simulink model "Aircraft_Simulator_full_long"  (R2024b)
settings: Solver=ode4  StartTime=0.0  StopTime=tfinal  FixedStep=dt  RelTol=1e-3
values from neighbouring files (symbols this model uses):
  A = [Xu  Xw  -w0  -9.81*cos(theta0) ... (first row only)    [Task3_code.m]
  A_long_period = [Xu+(w0*Zu)/(Zq+u0) -9.81*cos(theta0)-(w0*9.81*sin(theta0)/(Zq+u0)) ... (first row only)    [Task3_code.m]
  A_short_period = [Zw/(1-Zwd), (Zq+u0)/(1-Zwd) ... (first row only)    [Task3_code.m]
  aircraft_data = xlsread(filename_density_L, 'B2:B61')    [Task3_code.m]
  B = [Xde  Xdth ... (first row only)    [Task3_code.m]
  B_long_period = [Xde+(w0*Zde)/(Zq+u0) Xdth+(w0*Zdth)/(Zq+u0) ... (first row only)    [Task3_code.m]
  B_short_period = [Zde/(1-Zwd), Zdth/(1-Zwd) ... (first row only)    [Task3_code.m]
  C = eye(4,4)    [Task3_code.m]
  D = zeros(4,2)    [Task3_code.m]
  da = dc(1)    [Task3_code.m]
  de = 0    [Task3_code.m]
  dr = dc(2)    [Task3_code.m]
  dth = 10000    [Task3_code.m]
  F_gravity_0 = m*g * [ sin(s0(8)) ... (first row only)    [Task3_code.m]
  initial_conditions = [aircraft_data(13:15)' aircraft_data(10:12)' aircraft_data(4:6)' aircraft_data(7:9)' aircraft_data(18) aircraft_data(20) Vto 0]    [Task3_code.m]
  Ixx = aircraft_data(53)    [Task3_code.m]
  Iyy = aircraft_data(54)    [Task3_code.m]
  Izz = aircraft_data(55)    [Task3_code.m]
  m = aircraft_data(51)    [Task3_code.m]
  M0 = [0; 0; 0]    [Task3_code.m]
  s0 = aircraft_data(4:15)    [Task3_code.m]
undefined symbols (not defined in the file or in its folder): Matrix_Controls, Matrix_states
libraries: simulink_extras x8, shared6dof x1, aerolibasang x1
settings Model: Creator=yossef  LastModifiedBy=sheri
settings SolverCC: AlgebraicLoopSolver=TrustRegion
settings DataIOCC: ReturnWorkspaceOutputs=off
settings DebuggingCC: UnconnectedInputMsg=warning  UnconnectedOutputMsg=warning  UnconnectedLineMsg=warning  ArithmeticOperatorsInVariantConditions=warning
settings ModelReferenceCC: EnableRefExpFcnMdlSchedulingChecks=on
settings SFSimCC: SimUseLocalCustomCode=off  CustomCodeUndefinedFunction=UseInterfaceOnly
settings RTWCC: RTWUseLocalCustomCode=off  GPUComputeCapability=3.5

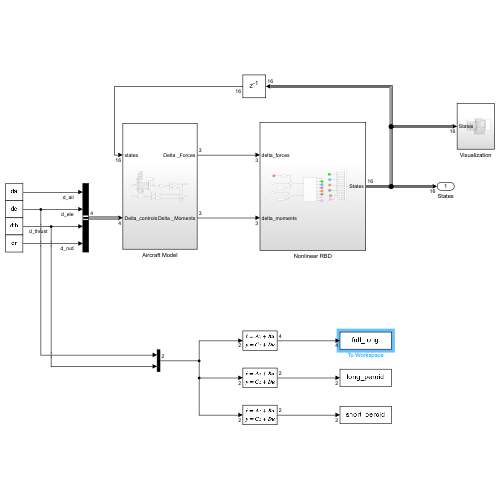
[thumbnail: Simulink's stored preview of the top-level diagram]
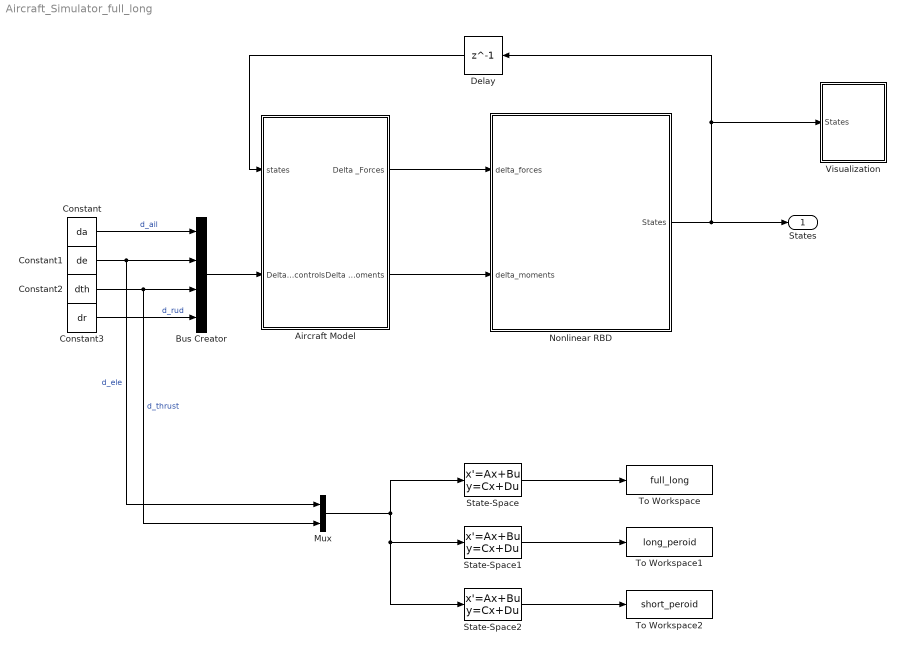
== system Aircraft_Simulator_full_long ==
  Aircraft Model : Subsystem
  Bus Creator : BusCreator  Inputs=4
  Constant : Constant  Value=da
  Constant1 : Constant  Value=de
  Constant2 : Constant  Value=dth
  Constant3 : Constant  Value=dr
  Delay : Delay  DelayLength=1  InitialCondition=initial_conditions
  Mux : Mux  Inputs=2
  Nonlinear RBD : Subsystem
  State-Space : StateSpace  A=A  B=B  C=C  D=D  InitialCondition=[s0(1),s0(3),s0(5),s0(8)]
  State-Space1 : StateSpace  A=A_long_period  B=B_long_period  C=eye(2,2)  D=zeros(2,2)  InitialCondition=[s0(1),s0(8)]
  State-Space2 : StateSpace  A=A_short_period  B=B_short_period  C=eye(2,2)  D=zeros(2,2)  InitialCondition=[aircraft_data(18),s0(5)]
  To Workspace : ToWorkspace  VariableName=full_long  SaveFormat=Timeseries  SampleTime=-1
  To Workspace1 : ToWorkspace  VariableName=long_peroid  SaveFormat=Timeseries  SampleTime=-1
  To Workspace2 : ToWorkspace  VariableName=short_peroid  SaveFormat=Timeseries  SampleTime=-1
  Visualization : Subsystem
  States : Outport
  wires:
  Delay/1 -> Aircraft Model/1(states)
  Nonlinear RBD/1(States) -> States/1, Delay/1, Visualization/1(States)
  Aircraft Model/1(Delta _Forces) -> Nonlinear RBD/1(delta_forces)
  Aircraft Model/2(Delta _Moments) -> Nonlinear RBD/2(delta_moments)
  Constant/1 -> Bus Creator/1  "d_ail"
  Constant1/1 -> Mux/1, Bus Creator/2  "d_ele"
  Constant2/1 -> Mux/2, Bus Creator/3  "d_thrust"
  Constant3/1 -> Bus Creator/4  "d_rud"
  Bus Creator/1 -> Aircraft Model/2(Delta_controls)
  Mux/1 -> State-Space/1, State-Space2/1, State-Space1/1
  State-Space/1 -> To Workspace/1
  State-Space2/1 -> To Workspace2/1
  State-Space1/1 -> To Workspace1/1

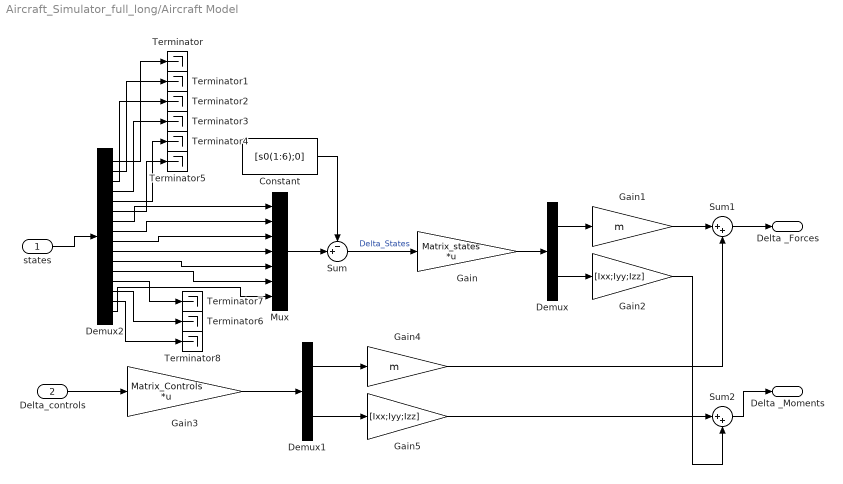
== system Aircraft_Simulator_full_long/Aircraft Model ==
  states : Inport
  Delta_controls : Inport  Port=2
  Constant : Constant  Value=[s0(1:6);0]
  Demux : Demux  Outputs=2
  Demux1 : Demux  Outputs=2
  Demux2 : Demux  Outputs=16
  Gain : Gain  Gain=Matrix_states  Multiplication=Matrix(K*u)
  Gain1 : Gain  Gain=m
  Gain2 : Gain  Gain=[Ixx;Iyy;Izz]
  Gain3 : Gain  Gain=Matrix_Controls  Multiplication=Matrix(K*u)
  Gain4 : Gain  Gain=m
  Gain5 : Gain  Gain=[Ixx;Iyy;Izz]
  Mux : Mux  Inputs=7
  Sum : Sum  Inputs=-+|
  Sum1 : Sum  Inputs=|++
  Sum2 : Sum  Inputs=|++
  Terminator{,1..8} (9 alike) : Terminator
  Delta _Forces : Outport
  Delta _Moments : Outport  Port=2
  wires:
  Mux/1 -> Sum/2
  Constant/1 -> Sum/1
  Sum/1 -> Gain/1  "Delta_States"
  Gain/1 -> Demux/1
  Demux/1 -> Gain1/1
  Demux/2 -> Gain2/1
  Gain2/1 -> Sum2/2
  Gain1/1 -> Sum1/1
  Sum1/1 -> Delta _Forces/1
  Sum2/1 -> Delta _Moments/1
  Delta_controls/1 -> Gain3/1
  Gain3/1 -> Demux1/1
  Demux1/1 -> Gain4/1
  Demux1/2 -> Gain5/1
  Gain4/1 -> Sum1/2
  Gain5/1 -> Sum2/1
  states/1 -> Demux2/1
  Demux2/1 -> Terminator/1
  Demux2/2 -> Terminator1/1
  Demux2/3 -> Terminator2/1
  Demux2/7 -> Mux/1
  Demux2/8 -> Mux/2
  Demux2/9 -> Mux/3
  Demux2/10 -> Mux/4
  Demux2/11 -> Mux/5
  Demux2/12 -> Mux/6
  Demux2/16 -> Mux/7
  Demux2/4 -> Terminator3/1
  Demux2/5 -> Terminator4/1
  Demux2/6 -> Terminator5/1
  Demux2/13 -> Terminator7/1
  Demux2/14 -> Terminator6/1
  Demux2/15 -> Terminator8/1

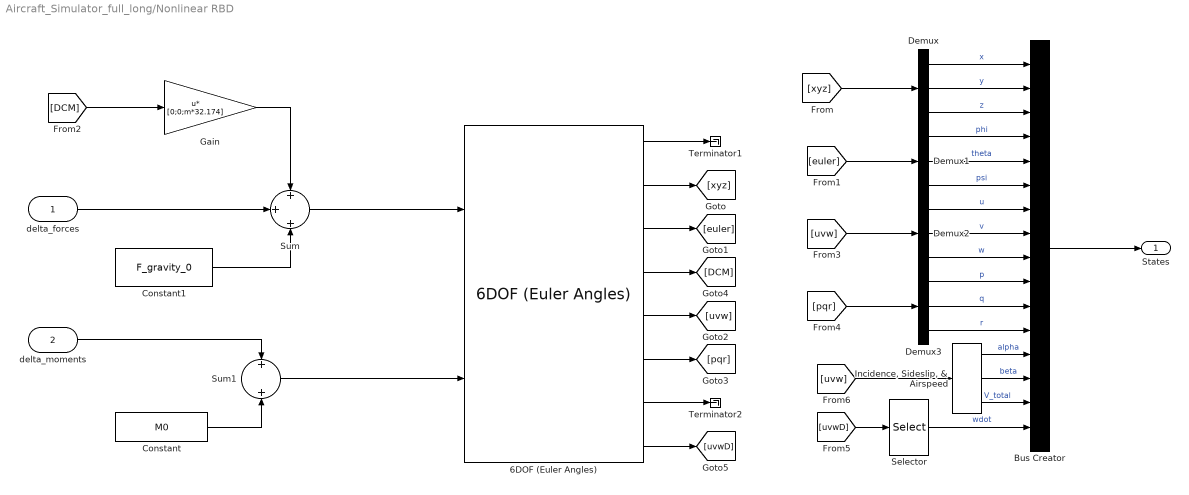
== system Aircraft_Simulator_full_long/Nonlinear RBD ==
  delta_forces : Inport
  delta_moments : Inport  Port=2
  6DOF (Euler Angles) : shared6dof/6DOF (Euler Angles)  units=English (Velocity in ft/s)  mtype=Fixed  rep=Euler Angles  xme_0=aircraft_data(13:15)  Vm_0=aircraft_data(4:6)  eul_0=aircraft_data(10:12)  pm_0=aircraft_data(7:9)  mass_0=m  mass_e=0.5  mass_f=2.0  inertia=I  inertia_e=eye(3)  inertia_f=2*eye(3)  k_quat=1.0  vre_flag=on  abi_flag=off  aMode=0  xme_statename=''  Vm_statename=''  eul_statename=''  quat_statename=''  pm_statename=''  mass_statename=''
  Bus Creator : BusCreator  Inputs=16
  Constant : Constant  Value=M0
  Constant1 : Constant  Value=F_gravity_0
  Demux{,1..3} (4 alike) : Demux  Outputs=3
  Gain : Gain  Gain=[0;0;m*32.174]  Multiplication=Matrix(u*K)
  "Incidence, Sideslip, & Airspeed" : aerolibasang/Incidence, Sideslip, & Airspeed
  Selector : Selector  InputPortWidth=3  IndexOptions=Index vector (dialog)  Indices=[3]  OutputSizes=1
  Sum : Sum  Inputs=+||+||+
  Sum1 : Sum  Inputs=+||+
  Terminator1 : Terminator
  Terminator2 : Terminator
  States : Outport
  wires:
  6DOF (Euler Angles)/4 -> [DCM]
  6DOF (Euler Angles)/1 -> Terminator1/1
  6DOF (Euler Angles)/2 -> [xyz]
  6DOF (Euler Angles)/3 -> [euler]
  6DOF (Euler Angles)/5 -> [uvw]
  6DOF (Euler Angles)/6 -> [pqr]
  6DOF (Euler Angles)/7 -> Terminator2/1
  6DOF (Euler Angles)/8 -> [uvwD]
  Demux/2 -> Bus Creator/2  "y"
  [xyz] -> Demux/1
  Demux/1 -> Bus Creator/1  "x"
  Demux/3 -> Bus Creator/3  "z"
  [uvw] -> Demux2/1
  [pqr] -> Demux3/1
  Demux1/1 -> Bus Creator/4  "phi"
  Demux1/2 -> Bus Creator/5  "theta"
  Demux1/3 -> Bus Creator/6  "psi"
  Demux2/1 -> Bus Creator/7  "u"
  Demux2/2 -> Bus Creator/8  "v"
  Demux2/3 -> Bus Creator/9  "w"
  Demux3/1 -> Bus Creator/10  "p"
  Demux3/2 -> Bus Creator/11  "q"
  Demux3/3 -> Bus Creator/12  "r"
  "Incidence, Sideslip, & Airspeed"/1 -> Bus Creator/13  "alpha"
  "Incidence, Sideslip, & Airspeed"/2 -> Bus Creator/14  "beta"
  "Incidence, Sideslip, & Airspeed"/3 -> Bus Creator/15  "V_total"
  [uvw] -> "Incidence, Sideslip, & Airspeed"/1
  Selector/1 -> Bus Creator/16  "wdot"
  [uvwD] -> Selector/1
  Bus Creator/1 -> States/1
  Constant1/1 -> Sum/3
  [DCM] -> Gain/1
  Gain/1 -> Sum/1
  Sum/1 -> 6DOF (Euler Angles)/1
  delta_forces/1 -> Sum/2
  Constant/1 -> Sum1/2
  delta_moments/1 -> Sum1/1
  Sum1/1 -> 6DOF (Euler Angles)/2
  [euler] -> Demux1/1

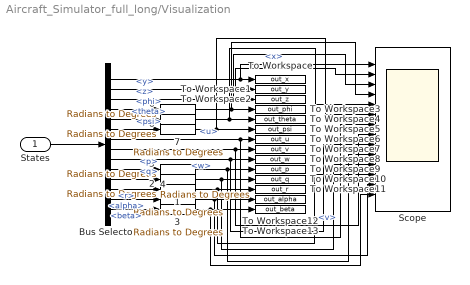
== system Aircraft_Simulator_full_long/Visualization ==
  States : Inport
  {1..8} (8 alike) : simulink_extras/Transformations/Radians to Degrees
  Bus Selector : BusSelector  OutputSignals=x,y,z,phi,theta,psi,u,v,w,p,q,r,alpha,beta
  Scope : Scope  NumInputPorts=14
  To Workspace : ToWorkspace  VariableName=out_x  SaveFormat=Timeseries  SampleTime=-1
  To Workspace1 : ToWorkspace  VariableName=out_y  SaveFormat=Timeseries  SampleTime=-1
  To Workspace10 : ToWorkspace  VariableName=out_q  SaveFormat=Timeseries  SampleTime=-1
  To Workspace11 : ToWorkspace  VariableName=out_r  SaveFormat=Timeseries  SampleTime=-1
  To Workspace12 : ToWorkspace  VariableName=out_alpha  SaveFormat=Timeseries  SampleTime=-1
  To Workspace13 : ToWorkspace  VariableName=out_beta  SaveFormat=Timeseries  SampleTime=-1
  To Workspace2 : ToWorkspace  VariableName=out_z  SaveFormat=Timeseries  SampleTime=-1
  To Workspace3 : ToWorkspace  VariableName=out_phi  SaveFormat=Timeseries  SampleTime=-1
  To Workspace4 : ToWorkspace  VariableName=out_theta  SaveFormat=Timeseries  SampleTime=-1
  To Workspace5 : ToWorkspace  VariableName=out_psi  SaveFormat=Timeseries  SampleTime=-1
  To Workspace6 : ToWorkspace  VariableName=out_u  SaveFormat=Timeseries  SampleTime=-1
  To Workspace7 : ToWorkspace  VariableName=out_v  SaveFormat=Timeseries  SampleTime=-1
  To Workspace8 : ToWorkspace  VariableName=out_w  SaveFormat=Timeseries  SampleTime=-1
  To Workspace9 : ToWorkspace  VariableName=out_p  SaveFormat=Timeseries  SampleTime=-1
  wires:
  States/1 -> Bus Selector/1
  Bus Selector/1 -> Scope/1, To Workspace/1  "<x>"
  Bus Selector/2 -> Scope/2, To Workspace1/1  "<y>"
  Bus Selector/3 -> Scope/3, To Workspace2/1  "<z>"
  Bus Selector/7 -> Scope/7, To Workspace6/1  "<u>"
  Bus Selector/8 -> Scope/8, To Workspace7/1  "<v>"
  Bus Selector/9 -> Scope/9, To Workspace8/1  "<w>"
  Bus Selector/11 -> 1/1  "<q>"
  1/1 -> Scope/11, To Workspace10/1
  Bus Selector/12 -> 2/1  "<r>"
  Bus Selector/13 -> 3/1  "<alpha>"
  Bus Selector/14 -> 4/1  "<beta>"
  4/1 -> Scope/14, To Workspace13/1
  3/1 -> Scope/13, To Workspace12/1
  2/1 -> Scope/12, To Workspace11/1
  Bus Selector/10 -> 5/1  "<p>"
  5/1 -> Scope/10, To Workspace9/1
  Bus Selector/4 -> 6/1  "<phi>"
  Bus Selector/5 -> 7/1  "<theta>"
  Bus Selector/6 -> 8/1  "<psi>"
  6/1 -> Scope/4, To Workspace3/1
  7/1 -> Scope/5, To Workspace4/1
  8/1 -> Scope/6, To Workspace5/1
